simulink model "simulacao_servo"  (R2017a)
settings: Solver=VariableStepAuto  StartTime=0.0  StopTime=60  RelTol=1e-3
settings Model: Creator=dscat  LastModifiedBy=dscat

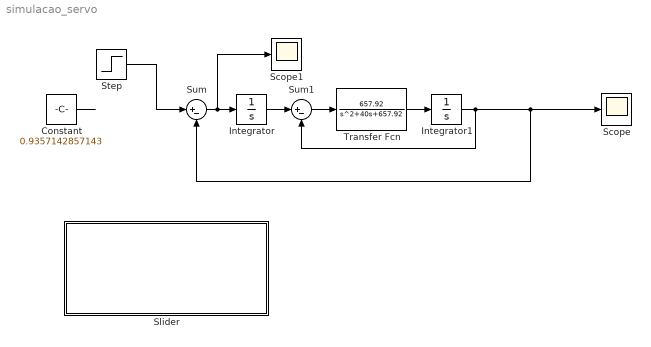
== system simulacao_servo ==
  Constant : Constant  Value=0.9357142857143
  Integrator : Integrator
  Integrator1 : Integrator
  Scope : Scope
  Scope1 : Scope
  Slider : Subsystem  DialogController=hmiCreateDDGDialog  IsWebBlock=on  mask(MWDashboardBlock){webBlockId=51c4cefd-a63e-407f-8103-2e00e04bd14c, webBlockType=slider, ShowInLibBrowser=on, ShowInitialText=on, HMISrcModelName=teste}
      mask prompts: webBlockId "WebBlock Id"; webBlockType "WebBlock Type"; HMISrcModelName "Source Model"
      mask help: SimulinkHMI:dialogs:SliderDialogDesc
      mask Help: helpview([docroot '/mapfiles/simulink.map'], 'hmi_slider')
      mask Display:
      | if strcmp(get_param(bdroot(gcb),'BlockDiagramType'), 'library')
      |     image([(matlabroot) '/toolbox/simulink/hmi/icons/Slider.png']);
      | end
  Step : Step  SampleTime=0
  Sum : Sum  Inputs=|+-
  Sum1 : Sum  Inputs=|+-
  Transfer Fcn : TransferFcn  Numerator=[657.92]  Denominator=[1 40 657.92]
  wires:
  Step/1 -> Sum/1
  Sum/1 -> Scope1/1, Integrator/1
  Integrator1/1 -> Sum/2, Scope/1, Sum1/2
  Transfer Fcn/1 -> Integrator1/1
  Integrator/1 -> Sum1/1
  Sum1/1 -> Transfer Fcn/1
  Constant/1 -> ?

== system simulacao_servo/Slider ==
